simulink model "PENDULUM_ACCEL_MODEL"  (R2025a)
settings: Solver=VariableStepAuto  StartTime=0.0  StopTime=10  RelTol=1e-3
values from neighbouring files (symbols this model uses):
  fs = 60    [PENDULUM_PARAMS.m]
  g = EstimatedParameters(5)    [PENDULUM_PARAMS.m]
  Ip = EstimatedParameters(3)    [PENDULUM_PARAMS.m]
  K = lqr(A, B, Q, R, N)    [PENDULUM_PARAMS.m]
  kt = EstimatedParameters(4)    [PENDULUM_PARAMS.m]
  measurement_variance = 1e-4    (= 0.0001)    [PENDULUM_PARAMS.m]
  mp = EstimatedParameters(2)    [PENDULUM_PARAMS.m]
  P0 = zeros(3, 3)    [PENDULUM_PARAMS.m]
  theta_0 = 10 * pi / 180    (= 0.174532925199)    [PENDULUM_PARAMS.m]
  theta_d_0 = 0    [PENDULUM_PARAMS.m]
  W = [7.5e-3,  0,    0 ... (first row only)    [PENDULUM_PARAMS.m]
  xp = EstimatedParameters(1)    [PENDULUM_PARAMS.m]
libraries: simulink_extras x4, simulink x1, slpidlib x1
settings Model: Creator=nyeff  LastModifiedBy=nyeff

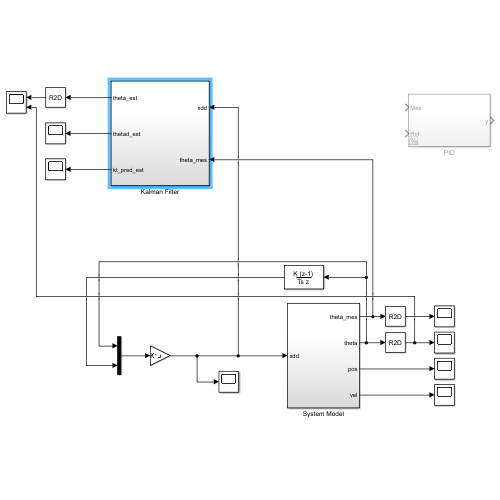
[thumbnail: Simulink's stored preview of the top-level diagram]
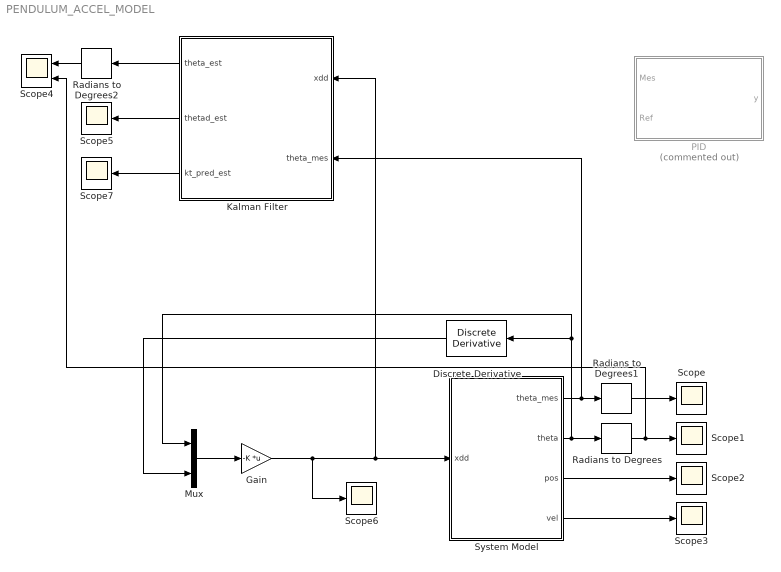
== system PENDULUM_ACCEL_MODEL ==
  Discrete Derivative : simulink/Discrete/Discrete Derivative  gainval=1.0  ICPrevScaledInput=0.0  OutMin=[]  OutMax=[]  OutDataType=fixdt(1, 16)  OutScaling=2^-10  DoSatur=off
  Gain : Gain  Gain=-K  Multiplication=Matrix(K*u)
  Kalman Filter : Subsystem
  Mux : Mux  Inputs=2
  PID : Subsystem  Commented=on
  Radians to Degrees : simulink_extras/Transformations/Radians to Degrees
  Radians to Degrees1 : simulink_extras/Transformations/Radians to Degrees
  Radians to Degrees2 : simulink_extras/Transformations/Radians to Degrees
  Scope{,1..3,5..7} (7 alike) : Scope
      Scope settings: ActiveDisplayYMinimum=25.762178364120928  ActiveDisplayYMaximum=55.840569459712881
      Scope1 settings: ActiveDisplayYMinimum=27.264963043982352  ActiveDisplayYMaximum=54.61533260415878
      Scope2 settings: ActiveDisplayYMinimum=-667.53299116997653  ActiveDisplayYMaximum=74.1703323522196  DataLoggingVariableName=ScopeData2
      Scope3 settings: ActiveDisplayYMinimum=-1.6636287913807664  ActiveDisplayYMaximum=0.18484764348675178  DataLoggingVariableName=ScopeData3
      Scope5 settings: ActiveDisplayYMinimum=-76.870856294383174  ActiveDisplayYMaximum=14.134154552837611  DataLoggingVariableName=ScopeData5
      Scope6 settings: ActiveDisplayYMinimum=-12.348876143899451  ActiveDisplayYMaximum=0.091869524278546777  DataLoggingVariableName=ScopeData6
      Scope7 settings: ActiveDisplayYMinimum=-0.0088285093642049631  ActiveDisplayYMaximum=0.079456584277844688  DataLoggingVariableName=ScopeData7
  Scope4 : Scope  NumInputPorts=2
      settings: ActiveDisplayYMinimum=-3.7417737113870313  ActiveDisplayYMaximum=12.268632447748416  DataLoggingVariableName=ScopeData4
  System Model : Subsystem
  wires:
  System Model/1(theta_mes) -> Kalman Filter/2(theta_mes), Radians to Degrees1/1
  System Model/2(theta) -> Discrete Derivative/1, Mux/1, Radians to Degrees/1
  Radians to Degrees/1 -> Scope4/2, Scope1/1
  Radians to Degrees1/1 -> Scope/1
  System Model/3(pos) -> Scope2/1
  System Model/4(vel) -> Scope3/1
  Kalman Filter/1(theta_est) -> Radians to Degrees2/1
  Kalman Filter/2(thetad_est) -> Scope5/1
  Radians to Degrees2/1 -> Scope4/1
  Mux/1 -> Gain/1
  Gain/1 -> Kalman Filter/1(xdd), System Model/1(xdd), Scope6/1
  Discrete Derivative/1 -> Mux/2
  Kalman Filter/3(kt_pred_est) -> Scope7/1

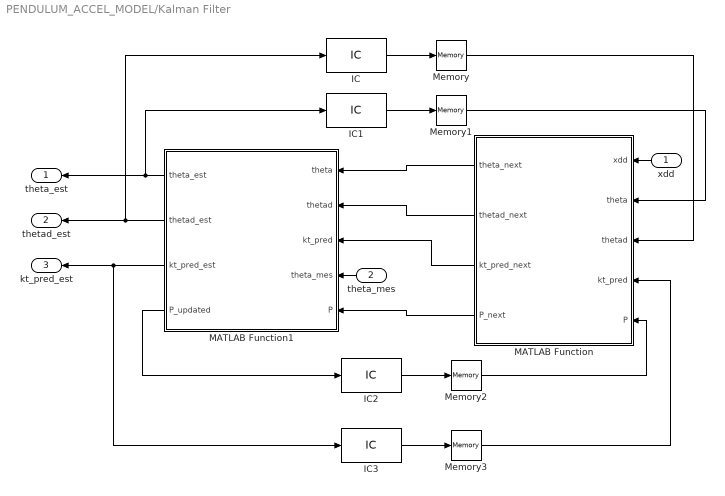
== system PENDULUM_ACCEL_MODEL/Kalman Filter ==
  xdd : Inport
  theta_mes : Inport  Port=2
  IC : InitialCondition  Value=theta_d_0
  IC1 : InitialCondition  Value=theta_0
  IC2 : InitialCondition  Value=P0
  IC3 : InitialCondition  Value=0
  MATLAB Function : MATLAB Function  TreatAsAtomicUnit=on
  MATLAB Function1 : MATLAB Function  TreatAsAtomicUnit=on
  Memory{,1..3} (4 alike) : Memory
  theta_est : Outport
  thetad_est : Outport  Port=2
  kt_pred_est : Outport  Port=3
  wires:
  xdd/1 -> MATLAB Function/1(xdd)
  MATLAB Function1/2(thetad_est) -> thetad_est/1, IC/1
  MATLAB Function/2(thetad_next) -> MATLAB Function1/2(thetad)
  MATLAB Function/1(theta_next) -> MATLAB Function1/1(theta)
  MATLAB Function/4(P_next) -> MATLAB Function1/5(P)
  theta_mes/1 -> MATLAB Function1/4(theta_mes)
  MATLAB Function1/4(P_updated) -> IC2/1
  Memory/1 -> MATLAB Function/3(thetad)
  Memory1/1 -> MATLAB Function/2(theta)
  IC/1 -> Memory/1
  IC1/1 -> Memory1/1
  Memory2/1 -> MATLAB Function/5(P)
  IC2/1 -> Memory2/1
  MATLAB Function1/1(theta_est) -> theta_est/1, IC1/1
  MATLAB Function/3(kt_pred_next) -> MATLAB Function1/3(kt_pred)
  MATLAB Function1/3(kt_pred_est) -> IC3/1, kt_pred_est/1
  IC3/1 -> Memory3/1
  Memory3/1 -> MATLAB Function/4(kt_pred)

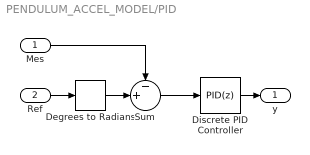
== system PENDULUM_ACCEL_MODEL/PID ==
  Mes : Inport
  Ref : Inport  Port=2
  Degrees to Radians : simulink_extras/Transformations/Degrees to Radians
  Discrete PID Controller : slpidlib/PID Controller  Controller=PID  Form=Parallel  TimeDomain=Discrete-time  UseExternalTs=off  SampleTime=-1  IntegratorMethod=Forward Euler  FilterMethod=Forward Euler  ControllerParametersSource=internal  P=37.7410232662455  I=68.1660056571599  UseKiTs=off  D=4.56194285385014  UseExternalDerivativeSource=off  N=115.84294097372  UseFilter=on  TunerSelectOption=Transfer Function Based (PID Tuner App)  InitialConditionSource=internal  InitialConditionForIntegrator=0  InitialConditionForFilter=0  DifferentiatorICPrevScaledInput=0  ExternalReset=none  TrackingMode=off  Kt=1  LimitOutput=off  SatLimitsSource=internal  UpperSaturationLimit=inf  LowerSaturationLimit=-inf  LinearizeAsGain=off  AntiWindupMode=none  Kb=1  LimitIntegrator=off  UpperIntegratorSaturationLimit=inf  LowerIntegratorSaturationLimit=-inf  POutMin=[]  POutMax=[]  IOutMin=[]  IOutMax=[]  DOutMin=[]  DOutMax=[]  NOutMin=[]  NOutMax=[]  SumOutMin=[]  SumOutMax=[]  SaturationOutMin=[]  SaturationOutMax=[]  PParamMin=[]  PParamMax=[]  IParamMin=[]  IParamMax=[]  DParamMin=[]  DParamMax=[]  NParamMin=[]  NParamMax=[]  KbParamMin=[]  KbParamMax=[]  KtParamMin=[]  KtParamMax=[]  KbOutMin=[]  KbOutMax=[]  KtOutMin=[]  KtOutMax=[]  IntegratorOutMin=[]  IntegratorOutMax=[]  FilterOutMin=[]  FilterOutMax=[]  SumI1OutMin=[]  SumI1OutMax=[]  SumI2OutMin=[]  SumI2OutMax=[]  SumI3OutMin=[]  SumI3OutMax=[]  SumI4OutMin=[]  SumI4OutMax=[]  SumDOutMin=[]  SumDOutMax=[]  DifferentiatorOutMin=[]  DifferentiatorOutMax=[]  FilterDiffOutCoefMin=[]  FilterDiffOutCoefMax=[]  ReciprocalOutMin=[]  ReciprocalOutMax=[]  SumDenOutMin=[]  SumDenOutMax=[]  SumNumOutMin=[]  SumNumOutMax=[]  DivideOutMin=[]  DivideOutMax=[]  UdiffTsProdOutMin=[]  UdiffTsProdOutMax=[]  NTsProdOutMin=[]  NTsProdOutMax=[]  UintegralTsProdOutMin=[]  UintegralTsProdOutMax=[]  UngainTsProdOutMin=[]  UngainTsProdOutMax=[]  ClampingZeroOutDataTypeStr=Inherit: Inherit via back propagation  ClampingZeroOutMin=[]  ClampingZeroOutMax=[]  FilterDenConstantOutDataTypeStr=Inherit: Inherit via back propagation  FilterDenConstantOutMin=[]  FilterDenConstantOutMax=[]  PCopyOutDataTypeStr=Inherit: Inherit via back propagation  PCopyOutMin=[]  PCopyOutMax=[]  NCopyOutDataTypeStr=Inherit: Inherit via back propagation  NCopyOutMin=[]  NCopyOutMax=[]  IntegratorContinuousStateAttributes=''  IntegratorStateMustResolveToSignalObject=off  IntegratorRTWStateStorageClass=Auto  FilterContinuousStateAttributes=''  FilterStateMustResolveToSignalObject=off  FilterRTWStateStorageClass=Auto  ParallelPVariant=InternalParameters  IdealPVariant=Disabled  IVariant=InternalParameters  DVariant=InternalParameters  IntegratorVariant=Discrete  SatVariant=Disabled  AWVariant=Passthrough  PCopyVariant=Disabled  TRVariant=Disabled  FdbkBlocksVariant=Forward  IdealPFdbkVariant=Disabled  SatFdbkVariant=Disabled  DerivativeFilterVariant=ForwardEulerFilter  NVariant=InternalParameters  NCopyVariant=Disabled  FilterICVariant=InternalICsFilter  IntegratorICVariant=InternalICs  ExternalResetVariant=Disabled  TRSumVariant=Passthrough  SumFdbkVariant=Disabled  SumVariant=Sum_PID  TsampFilterVariant=InternalTs  TsampNgainVariant=Passthrough  TsampIntegralVariant=Disabled_SignalSpec  ExternalSaturationOutDataTypeStr=Inherit: Same as second input  DerivativeSourceVariant=ErrorSignal  PreIntVariant=InternalPreInt
      settings: LibrarySourceBlock=simulink/Discrete/Discrete PID Controller
  Sum : Sum  Inputs=-+|
  y : Outport
  wires:
  Sum/1 -> Discrete PID Controller/1
  Mes/1 -> Sum/1
  Ref/1 -> Degrees to Radians/1
  Discrete PID Controller/1 -> y/1
  Degrees to Radians/1 -> Sum/2

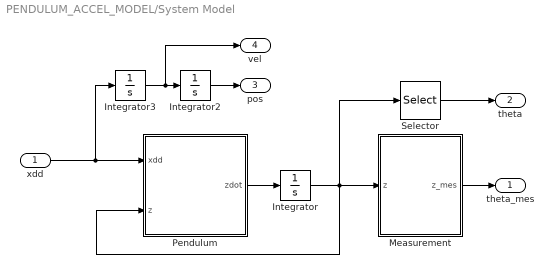
== system PENDULUM_ACCEL_MODEL/System Model ==
  xdd : Inport
  Integrator : Integrator  InitialCondition=[theta_0; theta_d_0]
  Integrator2 : Integrator  LimitOutput=on
  Integrator3 : Integrator
  Measurement : Subsystem
  Pendulum : Subsystem
  Selector : Selector  InputPortWidth=2  IndexOptions=Index vector (dialog)  Indices=[1]  OutputSizes=1
  theta_mes : Outport
  theta : Outport  Port=2
  pos : Outport  Port=3
  vel : Outport  Port=4
  wires:
  xdd/1 -> Pendulum/1(xdd), Integrator3/1
  Integrator2/1 -> pos/1
  Integrator3/1 -> vel/1, Integrator2/1
  Pendulum/1(zdot) -> Integrator/1
  Integrator/1 -> Measurement/1(z), Selector/1, Pendulum/2(z)
  Measurement/1(z_mes) -> theta_mes/1
  Selector/1 -> theta/1

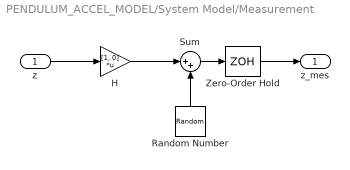
== system PENDULUM_ACCEL_MODEL/System Model/Measurement ==
  z : Inport
  H : Gain  Gain=[1, 0]  Multiplication=Matrix(K*u)
  Random Number : RandomNumber  Variance=measurement_variance  SampleTime=1/fs
  Sum : Sum  Inputs=|++
  Zero-Order Hold : ZeroOrderHold  SampleTime=1/fs
  z_mes : Outport
  wires:
  z/1 -> H/1
  Zero-Order Hold/1 -> z_mes/1
  Sum/1 -> Zero-Order Hold/1
  Random Number/1 -> Sum/2
  H/1 -> Sum/1

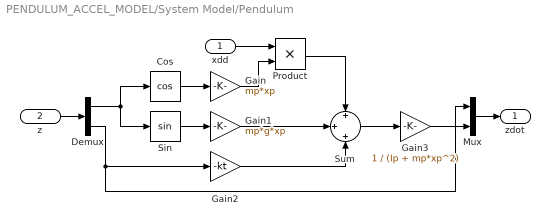
== system PENDULUM_ACCEL_MODEL/System Model/Pendulum ==
  xdd : Inport
  z : Inport  Port=2
  Cos : Trigonometry  Operator=cos
  Demux : Demux  Outputs=2
  Gain : Gain  Gain=mp*xp
  Gain1 : Gain  Gain=mp*g*xp
  Gain2 : Gain  Gain=-kt
  Gain3 : Gain  Gain=1 / (Ip + mp*xp^2)
  Mux : Mux  Inputs=2
  Product : Product
  Sin : Trigonometry
  Sum : Sum  Inputs=+|+|+
  zdot : Outport
  wires:
  xdd/1 -> Product/1
  Cos/1 -> Gain/1
  Gain/1 -> Product/2
  Sin/1 -> Gain1/1
  Gain1/1 -> Sum/2
  Gain2/1 -> Sum/3
  Product/1 -> Sum/1
  Sum/1 -> Gain3/1
  Demux/2 -> Gain2/1, Mux/1
  z/1 -> Demux/1
  Demux/1 -> Sin/1, Cos/1
  Gain3/1 -> Mux/2
  Mux/1 -> zdot/1

== matlab function PENDULUM_ACCEL_MODEL/Kalman Filter/MATLAB Function ==
  data: xdd input; theta_next output; theta input; thetad input; kt_pred input; P input; mp parameter; Ip parameter; xp parameter; thetad_next output; kt_pred_next output; fs parameter; P_next output; W parameter
function [theta_next, thetad_next, kt_pred_next, P_next] = Kalman_Predict(xdd, theta, thetad, kt_pred, P, mp, Ip, xp, fs, W)

g = 9.81;

thetadd = 1 / (Ip + mp*xp^2) * (mp*xdd*xp*cos(theta) + mp*g*xp*sin(theta) - kt_pred*thetad);

theta_next = theta + thetad * 1 / fs;
thetad_next = thetad + thetadd * 1 / fs;
kt_pred_next = kt_pred;

F = 1 / (fs*(Ip + mp*xp^2)) * [         fs*(Ip + mp*xp^2),                (Ip + mp*xp^2),     0;
                               mp*xp*(g*cos(theta) - xdd*sin(theta)),       -kt_pred,      -thetad     
                                              0 ,                               0,     fs*(Ip + mp*xp^2)];

P_next = F*P*F' + W;

== matlab function PENDULUM_ACCEL_MODEL/Kalman Filter/MATLAB Function1 ==
  data: theta input; theta_est output; thetad input; kt_pred input; theta_mes input; P input; thetad_est output; kt_pred_est output; P_updated output; V parameter
function [theta_est, thetad_est, kt_pred_est, P_updated] = Kalman_Update(theta, thetad, kt_pred, theta_mes, P, V)

y = theta_mes-theta;

H = [1, 0, 0];

S = H*P*H' + V;

K = P*H'/S;

x_updated = [theta; thetad; kt_pred] + K*y;

theta_est = x_updated(1);
thetad_est = x_updated(2);
kt_pred_est = x_updated(3);

P_updated = P - K*S*K';
